simulink model "case8"  (R2024b)
settings: Solver=FixedStepAuto  StartTime=0  StopTime=1  FixedStep=1e-7  RelTol=1e-3
values from neighbouring files (symbols this model uses):
  SG_D_1_D = 0.01056    [IEEE9_case_parameters.m]    (also in case1_parameters.m; case2_parameters.m; case3_parameters.m; case4_parameters.m)
  SG_D_1_EnableSaturation = 0    [IEEE9_case_parameters.m]    (also in case1_parameters.m; case2_parameters.m; case3_parameters.m; case4_parameters.m)
  SG_D_1_f0 = 60    [IEEE9_case_parameters.m]    (also in case1_parameters.m; case2_parameters.m; case3_parameters.m; case4_parameters.m)
  SG_D_1_H = 7.5    [IEEE9_case_parameters.m]    (also in case1_parameters.m; case2_parameters.m; case3_parameters.m; case4_parameters.m)
  SG_D_1_K_A = 20    [IEEE9_case_parameters.m]    (also in case1_parameters.m; case2_parameters.m; case3_parameters.m; case4_parameters.m)
  SG_D_1_K_E = 1.000000e+1    (= 10)    [IEEE9_case_parameters.m]    (also in case1_parameters.m; case2_parameters.m; case3_parameters.m; case4_parameters.m)
  SG_D_1_K_F = 2.363    [IEEE9_case_parameters.m]    (also in case1_parameters.m; case2_parameters.m; case3_parameters.m; case4_parameters.m)
  SG_D_1_K_s = 0.5    [IEEE9_case_parameters.m]    (also in case1_parameters.m = 5; case2_parameters.m = 5; case3_parameters.m = 5; case4_parameters.m = 5)
  SG_D_1_R_a = 0.001088    [IEEE9_case_parameters.m]    (also in case1_parameters.m; case2_parameters.m; case3_parameters.m; case4_parameters.m)
  SG_D_1_S_A = 1    [IEEE9_case_parameters.m]    (also in case1_parameters.m; case2_parameters.m; case3_parameters.m; case4_parameters.m)
  SG_D_1_S_B = 0.103    [IEEE9_case_parameters.m]    (also in case1_parameters.m; case2_parameters.m; case3_parameters.m; case4_parameters.m)
  SG_D_1_S_N = 10.659857    [IEEE9_case_parameters.m]    (also in case1_parameters.m; case2_parameters.m; case3_parameters.m; case4_parameters.m)
  SG_D_1_SpeedPara = 200    [IEEE9_case_parameters.m]    (also in case1_parameters.m; case2_parameters.m; case3_parameters.m; case4_parameters.m)
  SG_D_1_T_0 = 0.720173    [IEEE9_case_parameters.m]    (also in case1_parameters.m = 0.755522; case2_parameters.m = 0.808931; case3_parameters.m = 0.869402; case4_parameters.m = 0.729316)
  SG_D_1_T_1 = 0.3    [IEEE9_case_parameters.m]    (also in case1_parameters.m; case2_parameters.m; case3_parameters.m; case4_parameters.m)
  SG_D_1_T_2 = 0.05    [IEEE9_case_parameters.m]    (also in case1_parameters.m; case2_parameters.m; case3_parameters.m; case4_parameters.m)
  SG_D_1_T_3 = 0.02    [IEEE9_case_parameters.m]    (also in case1_parameters.m; case2_parameters.m; case3_parameters.m; case4_parameters.m)
  SG_D_1_T_4 = 0.005    [IEEE9_case_parameters.m]    (also in case1_parameters.m; case2_parameters.m; case3_parameters.m; case4_parameters.m)
  SG_D_1_T_A = 0.02    [IEEE9_case_parameters.m]    (also in case1_parameters.m; case2_parameters.m; case3_parameters.m; case4_parameters.m)
  SG_D_1_T_dd = 8.000000e+0    (= 8)    [IEEE9_case_parameters.m]    (also in case1_parameters.m; case2_parameters.m; case3_parameters.m; case4_parameters.m)
  SG_D_1_T_ddd = 0.04    [IEEE9_case_parameters.m]    (also in case1_parameters.m; case2_parameters.m; case3_parameters.m; case4_parameters.m)
  SG_D_1_T_E = 0.314    [IEEE9_case_parameters.m]    (also in case1_parameters.m; case2_parameters.m; case3_parameters.m; case4_parameters.m)
  SG_D_1_T_F = 0.35    [IEEE9_case_parameters.m]    (also in case1_parameters.m; case2_parameters.m; case3_parameters.m; case4_parameters.m)
  SG_D_1_T_qd = 0.8    [IEEE9_case_parameters.m]    (also in case1_parameters.m; case2_parameters.m; case3_parameters.m; case4_parameters.m)
  SG_D_1_T_qdd = 0.02    [IEEE9_case_parameters.m]    (also in case1_parameters.m; case2_parameters.m; case3_parameters.m; case4_parameters.m)
  SG_D_1_T_speed = 0.1    [IEEE9_case_parameters.m]    (also in case1_parameters.m = 200; case2_parameters.m = 200; case3_parameters.m = 200; case4_parameters.m = 200)
  SG_D_1_T_w = 0.5    [IEEE9_case_parameters.m]    (also in case1_parameters.m; case2_parameters.m; case3_parameters.m; case4_parameters.m)
  SG_D_1_V_ref = 1.990276    [IEEE9_case_parameters.m]    (also in case1_parameters.m = 2.042296; case2_parameters.m = 2.051388; case3_parameters.m = 2.089584; case4_parameters.m = 2.01845)
  SG_D_1_w_ref = 376.991118    [IEEE9_case_parameters.m]    (also in case1_parameters.m; case2_parameters.m; case3_parameters.m; case4_parameters.m)
  SG_D_1_wb = 6.000000e+1    (= 60)    [IEEE9_case_parameters.m]    (also in case1_parameters.m; case2_parameters.m; case3_parameters.m; case4_parameters.m)
  SG_D_1_x_d = 1.9    [IEEE9_case_parameters.m]    (also in case1_parameters.m; case2_parameters.m; case3_parameters.m; case4_parameters.m)
  SG_D_1_x_dd = 0.302    [IEEE9_case_parameters.m]    (also in case1_parameters.m; case2_parameters.m; case3_parameters.m; case4_parameters.m)
  SG_D_1_x_ddd = 0.204    [IEEE9_case_parameters.m]    (also in case1_parameters.m; case2_parameters.m; case3_parameters.m; case4_parameters.m)
  SG_D_1_x_l = 0.05    [IEEE9_case_parameters.m]    (also in case1_parameters.m; case2_parameters.m; case3_parameters.m; case4_parameters.m)
  SG_D_1_x_q = 1.3    [IEEE9_case_parameters.m]    (also in case1_parameters.m; case2_parameters.m; case3_parameters.m; case4_parameters.m)
  SG_D_1_x_qd = 0.5    [IEEE9_case_parameters.m]    (also in case1_parameters.m; case2_parameters.m; case3_parameters.m; case4_parameters.m)
  SG_D_1_x_qdd = 0.3    [IEEE9_case_parameters.m]    (also in case1_parameters.m; case2_parameters.m; case3_parameters.m; case4_parameters.m)
  SG_D_2_D = 0.02    [IEEE9_case_parameters.m]    (also in case1_parameters.m; case2_parameters.m; case3_parameters.m; case4_parameters.m)
  SG_D_2_EnableSaturation = 0    [IEEE9_case_parameters.m]    (also in case1_parameters.m; case2_parameters.m; case3_parameters.m; case4_parameters.m)
  SG_D_2_f0 = 60    [IEEE9_case_parameters.m]    (also in case1_parameters.m; case2_parameters.m; case3_parameters.m; case4_parameters.m)
  SG_D_2_H = 8.000000e+0    (= 8)    [IEEE9_case_parameters.m]    (also in case1_parameters.m; case2_parameters.m; case3_parameters.m; case4_parameters.m)
  SG_D_2_K_A = 20    [IEEE9_case_parameters.m]    (also in case1_parameters.m; case2_parameters.m; case3_parameters.m; case4_parameters.m)
  SG_D_2_K_E = 1.000000e+1    (= 10)    [IEEE9_case_parameters.m]    (also in case1_parameters.m; case2_parameters.m; case3_parameters.m; case4_parameters.m)
  SG_D_2_K_F = 2.363    [IEEE9_case_parameters.m]    (also in case1_parameters.m; case2_parameters.m; case3_parameters.m; case4_parameters.m)
  SG_D_2_K_s = 0.5    [IEEE9_case_parameters.m]    (also in case1_parameters.m = 4; case2_parameters.m = 4; case3_parameters.m = 4; case4_parameters.m = 4)
  SG_D_2_R_a = 0.001088    [IEEE9_case_parameters.m]    (also in case1_parameters.m; case2_parameters.m; case3_parameters.m; case4_parameters.m)
  SG_D_2_S_A = 1    [IEEE9_case_parameters.m]    (also in case1_parameters.m; case2_parameters.m; case3_parameters.m; case4_parameters.m)
  SG_D_2_S_B = 0.103    [IEEE9_case_parameters.m]    (also in case1_parameters.m; case2_parameters.m; case3_parameters.m; case4_parameters.m)
  SG_D_2_S_N = 10.659857    [IEEE9_case_parameters.m]    (also in case1_parameters.m; case2_parameters.m; case3_parameters.m; case4_parameters.m)
  SG_D_2_SpeedPara = 200    [IEEE9_case_parameters.m]    (also in case1_parameters.m; case2_parameters.m; case3_parameters.m; case4_parameters.m)
  SG_D_2_T_0 = 1.632913    [IEEE9_case_parameters.m]    (also in case1_parameters.m = 1.632925; case2_parameters.m = 1.632915; case3_parameters.m = 1.632914; case4_parameters.m = 1.632927)
  SG_D_2_T_1 = 0.2    [IEEE9_case_parameters.m]    (also in case1_parameters.m; case2_parameters.m; case3_parameters.m; case4_parameters.m)
  SG_D_2_T_2 = 0.05    [IEEE9_case_parameters.m]    (also in case1_parameters.m; case2_parameters.m; case3_parameters.m; case4_parameters.m)
  SG_D_2_T_3 = 0.02    [IEEE9_case_parameters.m]    (also in case1_parameters.m; case2_parameters.m; case3_parameters.m; case4_parameters.m)
  SG_D_2_T_4 = 0.005    [IEEE9_case_parameters.m]    (also in case1_parameters.m; case2_parameters.m; case3_parameters.m; case4_parameters.m)
  SG_D_2_T_A = 0.02    [IEEE9_case_parameters.m]    (also in case1_parameters.m; case2_parameters.m; case3_parameters.m; case4_parameters.m)
  SG_D_2_T_dd = 7.9    [IEEE9_case_parameters.m]    (also in case1_parameters.m; case2_parameters.m; case3_parameters.m; case4_parameters.m)
  SG_D_2_T_ddd = 0.04    [IEEE9_case_parameters.m]    (also in case1_parameters.m; case2_parameters.m; case3_parameters.m; case4_parameters.m)
  SG_D_2_T_E = 0.314    [IEEE9_case_parameters.m]    (also in case1_parameters.m; case2_parameters.m; case3_parameters.m; case4_parameters.m)
  SG_D_2_T_F = 0.35    [IEEE9_case_parameters.m]    (also in case1_parameters.m; case2_parameters.m; case3_parameters.m; case4_parameters.m)
  SG_D_2_T_qd = 0.8    [IEEE9_case_parameters.m]    (also in case1_parameters.m; case2_parameters.m; case3_parameters.m; case4_parameters.m)
  SG_D_2_T_qdd = 0.015    [IEEE9_case_parameters.m]    (also in case1_parameters.m; case2_parameters.m; case3_parameters.m; case4_parameters.m)
  SG_D_2_T_speed = 0.1    [IEEE9_case_parameters.m]    (also in case1_parameters.m = 150; case2_parameters.m = 150; case3_parameters.m = 150; case4_parameters.m = 150)
  SG_D_2_T_w = 0.35    [IEEE9_case_parameters.m]    (also in case1_parameters.m; case2_parameters.m; case3_parameters.m; case4_parameters.m)
  SG_D_2_V_ref = 2.58547    [IEEE9_case_parameters.m]    (also in case1_parameters.m = 2.597896; case2_parameters.m = 2.587136; case3_parameters.m = 2.586042; case4_parameters.m = 2.599679)
  SG_D_2_w_ref = 376.991118    [IEEE9_case_parameters.m]    (also in case1_parameters.m; case2_parameters.m; case3_parameters.m; case4_parameters.m)
  SG_D_2_wb = 6.000000e+1    (= 60)    [IEEE9_case_parameters.m]    (also in case1_parameters.m; case2_parameters.m; case3_parameters.m; case4_parameters.m)
  SG_D_2_x_d = 1.8    [IEEE9_case_parameters.m]    (also in case1_parameters.m; case2_parameters.m; case3_parameters.m; case4_parameters.m)
  SG_D_2_x_dd = 0.302    [IEEE9_case_parameters.m]    (also in case1_parameters.m; case2_parameters.m; case3_parameters.m; case4_parameters.m)
  SG_D_2_x_ddd = 0.204    [IEEE9_case_parameters.m]    (also in case1_parameters.m; case2_parameters.m; case3_parameters.m; case4_parameters.m)
  SG_D_2_x_l = 0.05    [IEEE9_case_parameters.m]    (also in case1_parameters.m; case2_parameters.m; case3_parameters.m; case4_parameters.m)
  SG_D_2_x_q = 1.25    [IEEE9_case_parameters.m]    (also in case1_parameters.m; case2_parameters.m; case3_parameters.m; case4_parameters.m)
  SG_D_2_x_qd = 0.5    [IEEE9_case_parameters.m]    (also in case1_parameters.m; case2_parameters.m; case3_parameters.m; case4_parameters.m)
  SG_D_2_x_qdd = 0.3    [IEEE9_case_parameters.m]    (also in case1_parameters.m; case2_parameters.m; case3_parameters.m; case4_parameters.m)
  SG_D_3_D = 0.02    [IEEE9_case_parameters.m]    (also in case1_parameters.m; case2_parameters.m; case3_parameters.m; case4_parameters.m)
  SG_D_3_EnableSaturation = 0    [IEEE9_case_parameters.m]    (also in case1_parameters.m; case2_parameters.m; case3_parameters.m; case4_parameters.m)
  SG_D_3_f0 = 60    [IEEE9_case_parameters.m]    (also in case1_parameters.m; case2_parameters.m; case3_parameters.m; case4_parameters.m)
  SG_D_3_H = 7.7    [IEEE9_case_parameters.m]    (also in case1_parameters.m; case2_parameters.m; case3_parameters.m; case4_parameters.m)
  SG_D_3_K_A = 20    [IEEE9_case_parameters.m]    (also in case1_parameters.m; case2_parameters.m; case3_parameters.m; case4_parameters.m)
  SG_D_3_K_E = 1.000000e+1    (= 10)    [IEEE9_case_parameters.m]    (also in case1_parameters.m; case2_parameters.m; case3_parameters.m; case4_parameters.m)
  SG_D_3_K_F = 2.363    [IEEE9_case_parameters.m]    (also in case1_parameters.m; case2_parameters.m; case3_parameters.m; case4_parameters.m)
  SG_D_3_K_s = 0.2    [IEEE9_case_parameters.m]    (also in case1_parameters.m = 2; case2_parameters.m = 2; case3_parameters.m = 2; case4_parameters.m = 2)
  SG_D_3_R_a = 0.001088    [IEEE9_case_parameters.m]    (also in case1_parameters.m; case2_parameters.m; case3_parameters.m; case4_parameters.m)
  SG_D_3_S_A = 1    [IEEE9_case_parameters.m]    (also in case1_parameters.m; case2_parameters.m; case3_parameters.m; case4_parameters.m)
  SG_D_3_S_B = 0.103    [IEEE9_case_parameters.m]    (also in case1_parameters.m; case2_parameters.m; case3_parameters.m; case4_parameters.m)
  SG_D_3_S_N = 10.659857    [IEEE9_case_parameters.m]    (also in case1_parameters.m; case2_parameters.m; case3_parameters.m; case4_parameters.m)
  SG_D_3_SpeedPara = 200    [IEEE9_case_parameters.m]    (also in case1_parameters.m; case2_parameters.m; case3_parameters.m; case4_parameters.m)
  SG_D_3_T_0 = 0.850788    [IEEE9_case_parameters.m]    (also in case1_parameters.m = 0.850786; case2_parameters.m = 0.850787; case3_parameters.m; case4_parameters.m = 0.850786)
  SG_D_3_T_1 = 0.2    [IEEE9_case_parameters.m]    (also in case1_parameters.m; case2_parameters.m; case3_parameters.m; case4_parameters.m)
  SG_D_3_T_2 = 0.05    [IEEE9_case_parameters.m]    (also in case1_parameters.m; case2_parameters.m; case3_parameters.m; case4_parameters.m)
  SG_D_3_T_3 = 0.02    [IEEE9_case_parameters.m]    (also in case1_parameters.m; case2_parameters.m; case3_parameters.m; case4_parameters.m)
  SG_D_3_T_4 = 0.005    [IEEE9_case_parameters.m]    (also in case1_parameters.m; case2_parameters.m; case3_parameters.m; case4_parameters.m)
  SG_D_3_T_A = 0.02    [IEEE9_case_parameters.m]    (also in case1_parameters.m; case2_parameters.m; case3_parameters.m; case4_parameters.m)
  SG_D_3_T_dd = 8.1    [IEEE9_case_parameters.m]    (also in case1_parameters.m; case2_parameters.m; case3_parameters.m; case4_parameters.m)
  SG_D_3_T_ddd = 0.04    [IEEE9_case_parameters.m]    (also in case1_parameters.m; case2_parameters.m; case3_parameters.m; case4_parameters.m)
  SG_D_3_T_E = 0.314    [IEEE9_case_parameters.m]    (also in case1_parameters.m; case2_parameters.m; case3_parameters.m; case4_parameters.m)
  SG_D_3_T_F = 0.35    [IEEE9_case_parameters.m]    (also in case1_parameters.m; case2_parameters.m; case3_parameters.m; case4_parameters.m)
  SG_D_3_T_qd = 0.8    [IEEE9_case_parameters.m]    (also in case1_parameters.m; case2_parameters.m; case3_parameters.m; case4_parameters.m)
  SG_D_3_T_qdd = 0.015    [IEEE9_case_parameters.m]    (also in case1_parameters.m; case2_parameters.m; case3_parameters.m; case4_parameters.m)
  SG_D_3_T_speed = 0.1    [IEEE9_case_parameters.m]    (also in case1_parameters.m = 180; case2_parameters.m = 180; case3_parameters.m = 180; case4_parameters.m = 180)
  SG_D_3_T_w = 0.4    [IEEE9_case_parameters.m]    (also in case1_parameters.m; case2_parameters.m; case3_parameters.m; case4_parameters.m)
  SG_D_3_V_ref = 1.892727    [IEEE9_case_parameters.m]    (also in case1_parameters.m = 1.906439; case2_parameters.m = 1.895535; case3_parameters.m = 1.892105; case4_parameters.m = 1.906598)
  SG_D_3_w_ref = 376.991118    [IEEE9_case_parameters.m]    (also in case1_parameters.m; case2_parameters.m; case3_parameters.m; case4_parameters.m)
  SG_D_3_wb = 6.000000e+1    (= 60)    [IEEE9_case_parameters.m]    (also in case1_parameters.m; case2_parameters.m; case3_parameters.m; case4_parameters.m)
  SG_D_3_x_d = 1.85    [IEEE9_case_parameters.m]    (also in case1_parameters.m; case2_parameters.m; case3_parameters.m; case4_parameters.m)
  SG_D_3_x_dd = 0.302    [IEEE9_case_parameters.m]    (also in case1_parameters.m; case2_parameters.m; case3_parameters.m; case4_parameters.m)
  SG_D_3_x_ddd = 0.204    [IEEE9_case_parameters.m]    (also in case1_parameters.m; case2_parameters.m; case3_parameters.m; case4_parameters.m)
  SG_D_3_x_l = 0.05    [IEEE9_case_parameters.m]    (also in case1_parameters.m; case2_parameters.m; case3_parameters.m; case4_parameters.m)
  SG_D_3_x_q = 1.2    [IEEE9_case_parameters.m]    (also in case1_parameters.m; case2_parameters.m; case3_parameters.m; case4_parameters.m)
  SG_D_3_x_qd = 0.5    [IEEE9_case_parameters.m]    (also in case1_parameters.m; case2_parameters.m; case3_parameters.m; case4_parameters.m)
  SG_D_3_x_qdd = 0.3    [IEEE9_case_parameters.m]    (also in case1_parameters.m; case2_parameters.m; case3_parameters.m; case4_parameters.m)
(part 6 of 12)

== system case8/SG_D_1/d_psi_kq_SG_D_1_block ==
  note: d_psi_kq_SG_D_1 in case8
      | $-\frac{\psi _{\mathrm{gq},\mathrm{SG},D,1}+\psi _{\mathrm{kq},\mathrm{SG},D,1}+\frac{\left(x_{l}-x_{\mathrm{qd}}\right)\,\left(\psi _{q,\mathrm{SG},D,1}+\frac{\psi _{\mathrm{gq},\mathrm{SG},D,1}\,\left(x_{l}-x_{\mathrm{qdd}}\right)}{x_{l}-x_{\mathrm{qd}}}+\frac{\psi _{\mathrm{kq},\mathrm{SG},D,1}\,\left(x_{\mathrm{qd}}-x_{\mathrm{qdd}}\right)}{x_{l}-x_{\mathrm{qd}}}\right)}{x_{\mathrm{qdd}}}}{T_{\mathrm{qdd}}}$
      | Automatically generated on 2025-10-31 19:29:35 .
  State_psi_gq_SG_D_1_da5e1 : Inport
  State_psi_kq_SG_D_1_411eb : Inport  Port=2
  State_psi_gq_SG_D_1_e86a4 : Inport  Port=3
  State_psi_kq_SG_D_1_1418e : Inport  Port=4
  State_psi_q_SG_D_1_82c28 : Inport  Port=5
  Add_44a13 : Sum
  Add_4c06f : Sum
  Add_520e3 : Sum
  Add_ae062 : Sum
  Add_d3269 : Sum
  Add_e20c1 : Sum
  Constant_-1_80ff6 : Constant  Value=-1
  Constant_-1_94d95 : Constant  Value=-1
  Constant_-1_9b79f : Constant  Value=-1
  Constant_-1_c1a20 : Constant  Value=-1
  Constant_-1_d85b0 : Constant  Value=-1
  Constant_T_qdd_9f64f : Constant  Value=T_qdd
  Constant_x_l_582b3 : Constant  Value=x_l
  Constant_x_l_8869d : Constant  Value=x_l
  Constant_x_l_cf13c : Constant  Value=x_l
  Constant_x_l_d8433 : Constant  Value=x_l
  Constant_x_qd_43f7a : Constant  Value=x_qd
  Constant_x_qd_a058d : Constant  Value=x_qd
  Constant_x_qd_df308 : Constant  Value=x_qd
  Constant_x_qd_e4029 : Constant  Value=x_qd
  Constant_x_qdd_14e66 : Constant  Value=x_qdd
  Constant_x_qdd_d1b96 : Constant  Value=x_qdd
  Constant_x_qdd_f1ee5 : Constant  Value=x_qdd
  Divide_0a53e : Product  Inputs=*/
  Divide_968ff : Product  Inputs=*/
  Divide_cdea9 : Product  Inputs=*/
  Divide_e4ae6 : Product  Inputs=*/
  Product_36f02 : Product
  Product_4a984 : Product
  Product_6fe3f : Product
  Product_7e6f7 : Product
  Product_834e3 : Product
  Product_86401 : Product
  Product_9f380 : Product
  Product_cd560 : Product
  Subtract_beb8c : Sum  Inputs=+-
  Subtract_ebc89 : Sum  Inputs=+-
  Subtract_fbb2e : Sum  Inputs=+-
  Blockout_d_psi_kq_SG_D_1_0e106 : Outport
  wires:
  Product_36f02/1 -> Add_e20c1/1
  Constant_-1_80ff6/1 -> Product_36f02/1
  Constant_x_l_d8433/1 -> Product_36f02/2
  Constant_x_qdd_f1ee5/1 -> Add_e20c1/2
  Constant_-1_c1a20/1 -> Product_6fe3f/1
  Constant_x_qd_df308/1 -> Subtract_fbb2e/1
  Constant_x_qd_e4029/1 -> Add_520e3/2
  Constant_-1_d85b0/1 -> Product_4a984/1
  Constant_x_l_cf13c/1 -> Product_6fe3f/2
  Constant_x_qdd_14e66/1 -> Subtract_fbb2e/2
  Constant_x_qd_43f7a/1 -> Add_ae062/2
  Constant_x_l_582b3/1 -> Product_4a984/2
  Subtract_beb8c/1 -> Add_d3269/1
  Product_7e6f7/1 -> Subtract_beb8c/1
  State_psi_gq_SG_D_1_e86a4/1 -> Product_86401/1
  Add_e20c1/1 -> Product_86401/2
  Product_4a984/1 -> Add_4c06f/1
  Constant_x_qd_a058d/1 -> Add_4c06f/2
  State_psi_kq_SG_D_1_1418e/1 -> Product_9f380/1
  Product_6fe3f/1 -> Add_ae062/1
  Subtract_fbb2e/1 -> Product_9f380/2
  Product_86401/1 -> Divide_968ff/1
  Add_4c06f/1 -> Divide_968ff/2
  Product_9f380/1 -> Divide_0a53e/1
  Add_ae062/1 -> Divide_0a53e/2
  Constant_-1_9b79f/1 -> Product_cd560/1
  Constant_x_l_8869d/1 -> Product_cd560/2
  Divide_968ff/1 -> Subtract_ebc89/1
  Divide_0a53e/1 -> Subtract_ebc89/2
  Product_cd560/1 -> Add_520e3/1
  Add_44a13/1 -> Product_834e3/2
  Subtract_ebc89/1 -> Add_44a13/1
  State_psi_q_SG_D_1_82c28/1 -> Add_44a13/2
  Constant_-1_94d95/1 -> Product_7e6f7/1
  State_psi_gq_SG_D_1_da5e1/1 -> Product_7e6f7/2
  Divide_e4ae6/1 -> Add_d3269/2
  Product_834e3/1 -> Divide_e4ae6/1
  Add_520e3/1 -> Product_834e3/1
  State_psi_kq_SG_D_1_411eb/1 -> Subtract_beb8c/2
  Constant_x_qdd_d1b96/1 -> Divide_e4ae6/2
  Add_d3269/1 -> Divide_cdea9/1
  Constant_T_qdd_9f64f/1 -> Divide_cdea9/2
  Divide_cdea9/1 -> Blockout_d_psi_kq_SG_D_1_0e106/1

== system case8/SG_D_1/d_psi_q_SG_D_1_block ==
  note: d_psi_q_SG_D_1 in case8
      | $2\,\pi \,f_{0}\,\left(v_{d,\mathrm{SG},D,1}\,\cos\left(\theta _{\mathrm{SG},D,1}\right)+v_{q,\mathrm{SG},D,1}\,\sin\left(\theta _{\mathrm{SG},D,1}\right)-\frac{R_{a}\,\left(\psi _{q,\mathrm{SG},D,1}+\frac{\psi _{\mathrm{gq},\mathrm{SG},D,1}\,\left(x_{l}-x_{\mathrm{qdd}}\right)}{x_{l}-x_{\mathrm{qd}}}+\frac{\psi _{\mathrm{kq},\mathrm{SG},D,1}\,\left(x_{\mathrm{qd}}-x_{\mathrm{qdd}}\right)}{x_{l}-x_{\mathrm{qd}}}\right)}{x_{\mathrm{qdd}}}-\frac{\psi _{d,\mathrm{SG},D,1}\,w_{\mathrm{SG},D,1}}{2\,f_{0}\,\pi }\right)$
      | Automatically generated on 2025-10-31 19:29:30 .
  State_psi_gq_SG_D_1_7fe2e : Inport
  State_psi_kq_SG_D_1_b8294 : Inport  Port=2
  State_psi_q_SG_D_1_982cf : Inport  Port=3
  Input_v_d_SG_D_1_59a52 : Inport  Port=4
  State_theta_SG_D_1_06da5 : Inport  Port=5
  Input_v_q_SG_D_1_df1d2 : Inport  Port=6
  State_theta_SG_D_1_a61ef : Inport  Port=7
  State_psi_d_SG_D_1_9d031 : Inport  Port=8
  State_w_SG_D_1_bb027 : Inport  Port=9
  Add_5c444 : Sum
  Add_a27cd : Sum
  Add_c86fd : Sum
  Add_d6098 : Sum
  Add_ed7bc : Sum
  Constant_-1_06fe4 : Constant  Value=-1
  Constant_-1_09968 : Constant  Value=-1
  Constant_-1_faf80 : Constant  Value=-1
  Constant_-2.0_2267e : Constant  Value=-2.0
  Constant_2.0_87b9f : Constant  Value=2.0
  Constant_R_a_73440 : Constant  Value=R_a
  Constant_f0_32b31 : Constant  Value=f0
  Constant_f0_f8d6c : Constant  Value=f0
  Constant_pi_3286e : Constant  Value=pi
  Constant_pi_4e0a1 : Constant  Value=pi
  Constant_x_l_61a17 : Constant  Value=x_l
  Constant_x_l_a1f9c : Constant  Value=x_l
  Constant_x_l_f6918 : Constant  Value=x_l
  Constant_x_qd_0a3c7 : Constant  Value=x_qd
  Constant_x_qd_a448b : Constant  Value=x_qd
  Constant_x_qd_e83f7 : Constant  Value=x_qd
  Constant_x_qdd_2b385 : Constant  Value=x_qdd
  Constant_x_qdd_98a4f : Constant  Value=x_qdd
  Constant_x_qdd_9a601 : Constant  Value=x_qdd
  Divide_20893 : Product  Inputs=*/
  Divide_2ec5d : Product  Inputs=*/
  Divide_35f3f : Product  Inputs=*/
  Divide_dcf87 : Product  Inputs=*/
  MathFunc_cos_bd0e0 : Trigonometry  Operator=cos
  MathFunc_sin_a6dc1 : Trigonometry
  Product_019c9 : Product
  Product_2a58c : Product
  Product_2ca41 : Product
  Product_347ca : Product
  Product_486e4 : Product
  Product_88d0c : Product
  Product_acb5a : Product
  Product_b748f : Product
  Product_c36d3 : Product
  Product_c7bec : Product
  Product_d2a7c : Product
  Product_dd8ad : Product
  Product_eb19a : Product
  Product_ebe4b : Product
  Subtract_0ac44 : Sum  Inputs=+-
  Subtract_1ca24 : Sum  Inputs=+-
  Subtract_30cfb : Sum  Inputs=+-
  Subtract_b4afb : Sum  Inputs=+-
  Blockout_d_psi_q_SG_D_1_a9dc6 : Outport
  wires:
  Divide_35f3f/1 -> Subtract_b4afb/1
  Product_dd8ad/1 -> Add_d6098/1
  Constant_x_l_a1f9c/1 -> Product_dd8ad/2
  Constant_-1_09968/1 -> Product_dd8ad/1
  Constant_x_qdd_9a601/1 -> Add_d6098/2
  Constant_x_l_f6918/1 -> Product_2ca41/2
  Constant_-1_faf80/1 -> Product_2ca41/1
  Constant_x_l_61a17/1 -> Product_c7bec/2
  Constant_x_qdd_98a4f/1 -> Subtract_1ca24/2
  State_psi_kq_SG_D_1_b8294/1 -> Product_486e4/1
  Constant_-1_06fe4/1 -> Product_c7bec/1
  Constant_x_qd_0a3c7/1 -> Subtract_1ca24/1
  State_psi_gq_SG_D_1_7fe2e/1 -> Product_eb19a/1
  Product_347ca/1 -> Blockout_d_psi_q_SG_D_1_a9dc6/1
  Subtract_b4afb/1 -> Add_c86fd/1
  Product_eb19a/1 -> Divide_35f3f/1
  Add_d6098/1 -> Product_eb19a/2
  Divide_dcf87/1 -> Subtract_b4afb/2
  Product_2ca41/1 -> Add_ed7bc/1
  Constant_x_qd_a448b/1 -> Add_ed7bc/2
  Constant_-2.0_2267e/1 -> Product_2a58c/1
  Product_486e4/1 -> Divide_dcf87/1
  Product_c7bec/1 -> Add_a27cd/1
  Subtract_1ca24/1 -> Product_486e4/2
  Constant_x_qd_e83f7/1 -> Add_a27cd/2
  Add_ed7bc/1 -> Divide_35f3f/2
  Add_a27cd/1 -> Divide_dcf87/2
  Constant_f0_f8d6c/1 -> Product_ebe4b/2
  State_psi_q_SG_D_1_982cf/1 -> Add_c86fd/2
  Product_d2a7c/1 -> Product_c36d3/1
  Constant_R_a_73440/1 -> Product_b748f/1
  Product_c36d3/1 -> Divide_20893/2
  Product_b748f/1 -> Divide_2ec5d/1
  Add_c86fd/1 -> Product_b748f/2
  State_theta_SG_D_1_06da5/1 -> MathFunc_cos_bd0e0/1
  Input_v_d_SG_D_1_59a52/1 -> Product_019c9/1
  Constant_x_qdd_2b385/1 -> Divide_2ec5d/2
  MathFunc_cos_bd0e0/1 -> Product_019c9/2
  State_theta_SG_D_1_a61ef/1 -> MathFunc_sin_a6dc1/1
  Divide_2ec5d/1 -> Subtract_0ac44/1
  Constant_2.0_87b9f/1 -> Product_d2a7c/1
  State_w_SG_D_1_bb027/1 -> Product_acb5a/2
  Constant_pi_4e0a1/1 -> Product_d2a7c/2
  Subtract_30cfb/1 -> Add_5c444/1
  Product_019c9/1 -> Subtract_0ac44/2
  Divide_20893/1 -> Add_5c444/2
  Input_v_q_SG_D_1_df1d2/1 -> Product_88d0c/1
  MathFunc_sin_a6dc1/1 -> Product_88d0c/2
  Product_88d0c/1 -> Subtract_30cfb/2
  State_psi_d_SG_D_1_9d031/1 -> Product_acb5a/1
  Constant_f0_32b31/1 -> Product_c36d3/2
  Constant_pi_3286e/1 -> Product_2a58c/2
  Subtract_0ac44/1 -> Subtract_30cfb/1
  Product_acb5a/1 -> Divide_20893/1
  Product_2a58c/1 -> Product_ebe4b/1
  Product_ebe4b/1 -> Product_347ca/1
  Add_5c444/1 -> Product_347ca/2

== system case8/SG_D_1/d_theta_SG_D_1_block ==
  note: d_theta_SG_D_1 in case8
      | $w_{\mathrm{SG},D,1}-2\,\pi \,f_{0}$
      | Automatically generated on 2025-10-31 19:29:36 .
  State_w_SG_D_1_1d023 : Inport
  Add_d6c34 : Sum
  Constant_-2.0_1c6c2 : Constant  Value=-2.0
  Constant_f0_3bb0f : Constant  Value=f0
  Constant_pi_2d319 : Constant  Value=pi
  Product_4123a : Product
  Product_fbd34 : Product
  Blockout_d_theta_SG_D_1_4230e : Outport
  wires:
  State_w_SG_D_1_1d023/1 -> Add_d6c34/2
  Constant_-2.0_1c6c2/1 -> Product_4123a/1
  Constant_f0_3bb0f/1 -> Product_fbd34/2
  Constant_pi_2d319/1 -> Product_4123a/2
  Product_fbd34/1 -> Add_d6c34/1
  Product_4123a/1 -> Product_fbd34/1
  Add_d6c34/1 -> Blockout_d_theta_SG_D_1_4230e/1

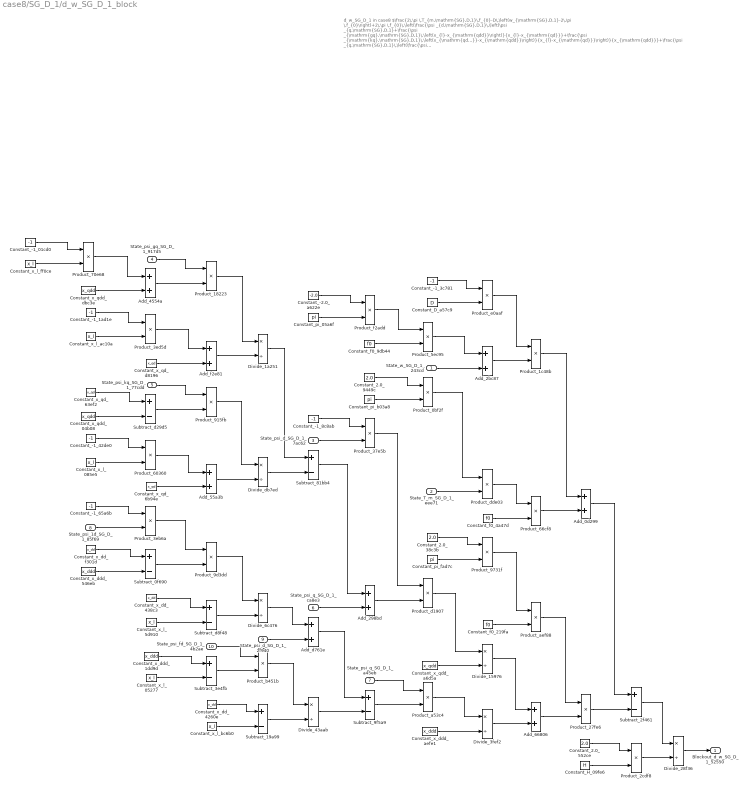
== system case8/SG_D_1/d_w_SG_D_1_block ==
  note: d_w_SG_D_1 in case8
      | $\frac{2\,\pi \,T_{m,\mathrm{SG},D,1}\,f_{0}-D\,\left(w_{\mathrm{SG},D,1}-2\,\pi \,f_{0}\right)+2\,\pi \,f_{0}\,\left(\frac{\psi _{d,\mathrm{SG},D,1}\,\left(\psi _{q,\mathrm{SG},D,1}+\frac{\psi _{\mathrm{gq},\mathrm{SG},D,1}\,\left(x_{l}-x_{\mathrm{qdd}}\right)}{x_{l}-x_{\mathrm{qd}}}+\frac{\psi _{\mathrm{kq},\mathrm{SG},D,1}\,\left(x_{\mathrm{qd}}-x_{\mathrm{qdd}}\right)}{x_{l}-x_{\mathrm{qd}}}\right)}{x_{\mathrm{qdd}}}+\frac{\psi _{q,\mathrm{SG},D,1}\,\left(\frac{\psi _{\mathrm{1d},\mathrm{SG},D,1}\,\left(x_{\mathrm{dd}}-x_{\mathrm{ddd}}\right)}{x_{\mathrm{dd}}-x_{l}}-\psi _{d,\mathrm{SG},D,1}+\frac{\psi _{\mathrm{fd},\mathrm{SG},D,1}\,\left(x_{\mathrm{ddd}}-x_{l}\right)}{x_{\mathrm{dd}}-x_{l}}\right)}{x_{\mathrm{ddd}}}\right)}{2\,H}$
      | Automatically generated on 2025-10-31 19:29:36 .
  State_w_SG_D_1_243cd : Inport
  State_T_m_SG_D_1_eee71 : Inport  Port=2
  State_psi_d_SG_D_1_7ac62 : Inport  Port=3
  State_psi_gq_SG_D_1_917d5 : Inport  Port=4
  State_psi_kq_SG_D_1_77cdd : Inport  Port=5
  State_psi_q_SG_D_1_ca8e3 : Inport  Port=6
  State_psi_q_SG_D_1_a45eb : Inport  Port=7
  State_psi_1d_SG_D_1_85f69 : Inport  Port=8
  State_psi_d_SG_D_1_2f940 : Inport  Port=9
  State_psi_fd_SG_D_1_4b2ae : Inport  Port=10
  Add_0d299 : Sum
  Add_298bd : Sum
  Add_2bc87 : Sum
  Add_4554a : Sum
  Add_55a3b : Sum
  Add_66806 : Sum
  Add_d761e : Sum
  Add_f2e81 : Sum
  Constant_-1_01cd0 : Constant  Value=-1
  Constant_-1_1ad1e : Constant  Value=-1
  Constant_-1_3c781 : Constant  Value=-1
  Constant_-1_42de0 : Constant  Value=-1
  Constant_-1_65a6b : Constant  Value=-1
  Constant_-1_8c8ab : Constant  Value=-1
  Constant_-2.0_a622e : Constant  Value=-2.0
  Constant_2.0_38c3b : Constant  Value=2.0
  Constant_2.0_552ce : Constant  Value=2.0
  Constant_2.0_9449c : Constant  Value=2.0
  Constant_D_a57c9 : Constant  Value=D
  Constant_H_09fe6 : Constant  Value=H
  Constant_f0_219fa : Constant  Value=f0
  Constant_f0_4a47d : Constant  Value=f0
  Constant_f0_9db44 : Constant  Value=f0
  Constant_pi_05a6f : Constant  Value=pi
  Constant_pi_b03a8 : Constant  Value=pi
  Constant_pi_fad7c : Constant  Value=pi
  Constant_x_dd_4260e : Constant  Value=x_dd
  Constant_x_dd_438c3 : Constant  Value=x_dd
  Constant_x_dd_f301d : Constant  Value=x_dd
  Constant_x_ddd_1dd9d : Constant  Value=x_ddd
  Constant_x_ddd_546eb : Constant  Value=x_ddd
  Constant_x_ddd_aefe1 : Constant  Value=x_ddd
  Constant_x_l_05277 : Constant  Value=x_l
  Constant_x_l_085e5 : Constant  Value=x_l
  Constant_x_l_5d910 : Constant  Value=x_l
  Constant_x_l_ac10a : Constant  Value=x_l
  Constant_x_l_bc6b0 : Constant  Value=x_l
  Constant_x_l_ff0ce : Constant  Value=x_l
  Constant_x_qd_63ef2 : Constant  Value=x_qd
  Constant_x_qd_6b94e : Constant  Value=x_qd
  Constant_x_qd_d8196 : Constant  Value=x_qd
  Constant_x_qdd_04b08 : Constant  Value=x_qdd
  Constant_x_qdd_a6d5a : Constant  Value=x_qdd
  Constant_x_qdd_dbc3e : Constant  Value=x_qdd
  Divide_15976 : Product  Inputs=*/
  Divide_1a251 : Product  Inputs=*/
  Divide_28f36 : Product  Inputs=*/
  Divide_3fef2 : Product  Inputs=*/
  Divide_43aab : Product  Inputs=*/
  Divide_6c476 : Product  Inputs=*/
  Divide_db7ed : Product  Inputs=*/
  Product_0bf2f : Product
  Product_18223 : Product
  Product_1c48b : Product
  Product_27fe6 : Product
  Product_2cdf8 : Product
  Product_37e5b : Product
  Product_3eb6a : Product
  Product_3ed5d : Product
  Product_5ec95 : Product
  Product_60360 : Product
  Product_66cf8 : Product
  Product_70e68 : Product
  Product_915fb : Product
  Product_9731f : Product
  Product_9d3dd : Product
  Product_a53c4 : Product
  Product_aef88 : Product
  Product_b451b : Product
  Product_d1907 : Product
  Product_dde03 : Product
  Product_e0aaf : Product
  Product_f2add : Product
  Subtract_0f690 : Sum  Inputs=+-
  Subtract_19a99 : Sum  Inputs=+-
  Subtract_2f461 : Sum  Inputs=+-
  Subtract_3e4fb : Sum  Inputs=+-
  Subtract_81bb4 : Sum  Inputs=+-
  Subtract_9f5a9 : Sum  Inputs=+-
  Subtract_d29d5 : Sum  Inputs=+-
  Subtract_d8f48 : Sum  Inputs=+-
  Blockout_d_w_SG_D_1_52550 : Outport
  wires:
  Product_5ec95/1 -> Add_2bc87/1
  Constant_-1_01cd0/1 -> Product_70e68/1
  Constant_pi_b03a8/1 -> Product_0bf2f/2
  Constant_x_qdd_dbc3e/1 -> Add_4554a/2
  Constant_x_l_ff0ce/1 -> Product_70e68/2
  Product_70e68/1 -> Add_4554a/1
  Constant_x_qd_63ef2/1 -> Subtract_d29d5/1
  Constant_-1_1ad1e/1 -> Product_3ed5d/1
  Product_f2add/1 -> Product_5ec95/1
  Constant_x_qdd_04b08/1 -> Subtract_d29d5/2
  State_psi_q_SG_D_1_a45eb/1 -> Product_a53c4/1
  Constant_x_l_ac10a/1 -> Product_3ed5d/2
  Constant_-1_42de0/1 -> Product_60360/1
  Constant_x_l_085e5/1 -> Product_60360/2
  Constant_-1_65a6b/1 -> Product_3eb6a/1
  Product_3ed5d/1 -> Add_f2e81/1
  State_psi_1d_SG_D_1_85f69/1 -> Product_3eb6a/2
  Constant_x_dd_f301d/1 -> Subtract_0f690/1
  Subtract_d29d5/1 -> Product_915fb/2
  Constant_x_ddd_546eb/1 -> Subtract_0f690/2
  State_psi_gq_SG_D_1_917d5/1 -> Product_18223/1
  Product_37e5b/1 -> Product_d1907/1
  Add_4554a/1 -> Product_18223/2
  Constant_x_qd_d8196/1 -> Add_f2e81/2
  State_psi_kq_SG_D_1_77cdd/1 -> Product_915fb/1
  Constant_f0_9db44/1 -> Product_5ec95/2
  Product_60360/1 -> Add_55a3b/1
  Constant_x_dd_438c3/1 -> Subtract_d8f48/1
  Constant_x_qd_6b94e/1 -> Add_55a3b/2
  Product_3eb6a/1 -> Product_9d3dd/1
  Subtract_0f690/1 -> Product_9d3dd/2
  Constant_x_l_5d910/1 -> Subtract_d8f48/2
  Constant_x_ddd_1dd9d/1 -> Subtract_3e4fb/1
  Constant_x_l_05277/1 -> Subtract_3e4fb/2
  State_w_SG_D_1_243cd/1 -> Add_2bc87/2
  Divide_15976/1 -> Add_66806/1
  Constant_-1_3c781/1 -> Product_e0aaf/1
  Product_18223/1 -> Divide_1a251/1
  Add_2bc87/1 -> Product_1c48b/2
  Divide_1a251/1 -> Subtract_81bb4/1
  Add_f2e81/1 -> Divide_1a251/2
  Constant_pi_05a6f/1 -> Product_f2add/2
  Product_915fb/1 -> Divide_db7ed/1
  Add_55a3b/1 -> Divide_db7ed/2
  Product_9d3dd/1 -> Divide_6c476/1
  Divide_6c476/1 -> Add_d761e/1
  Subtract_d8f48/1 -> Divide_6c476/2
  State_psi_fd_SG_D_1_4b2ae/1 -> Product_b451b/1
  Subtract_3e4fb/1 -> Product_b451b/2
  Constant_x_dd_4260e/1 -> Subtract_19a99/1
  Constant_x_l_bc6b0/1 -> Subtract_19a99/2
  Divide_db7ed/1 -> Subtract_81bb4/2
  Constant_2.0_9449c/1 -> Product_0bf2f/1
  State_psi_d_SG_D_1_2f940/1 -> Add_d761e/2
  Product_b451b/1 -> Divide_43aab/1
  Subtract_19a99/1 -> Divide_43aab/2
  Constant_-2.0_a622e/1 -> Product_f2add/1
  Constant_-1_8c8ab/1 -> Product_37e5b/1
  State_psi_d_SG_D_1_7ac62/1 -> Product_37e5b/2
  Subtract_81bb4/1 -> Add_298bd/1
  Subtract_9f5a9/1 -> Product_a53c4/2
  State_psi_q_SG_D_1_ca8e3/1 -> Add_298bd/2
  Add_d761e/1 -> Subtract_9f5a9/1
  Divide_43aab/1 -> Subtract_9f5a9/2
  Add_298bd/1 -> Product_d1907/2
  Constant_D_a57c9/1 -> Product_e0aaf/2
  Product_0bf2f/1 -> Product_dde03/1
  State_T_m_SG_D_1_eee71/1 -> Product_dde03/2
  Constant_2.0_38c3b/1 -> Product_9731f/1
  Constant_pi_fad7c/1 -> Product_9731f/2
  Product_d1907/1 -> Divide_15976/1
  Constant_x_qdd_a6d5a/1 -> Divide_15976/2
  Product_a53c4/1 -> Divide_3fef2/1
  Constant_x_ddd_aefe1/1 -> Divide_3fef2/2
  Product_e0aaf/1 -> Product_1c48b/1
  Product_dde03/1 -> Product_66cf8/1
  Constant_f0_4a47d/1 -> Product_66cf8/2
  Product_9731f/1 -> Product_aef88/1
  Constant_f0_219fa/1 -> Product_aef88/2
  Divide_3fef2/1 -> Add_66806/2
  Product_1c48b/1 -> Add_0d299/1
  Product_66cf8/1 -> Add_0d299/2
  Product_aef88/1 -> Product_27fe6/1
  Add_66806/1 -> Product_27fe6/2
  Add_0d299/1 -> Subtract_2f461/1
  Product_27fe6/1 -> Subtract_2f461/2
  Constant_2.0_552ce/1 -> Product_2cdf8/1
  Constant_H_09fe6/1 -> Product_2cdf8/2
  Subtract_2f461/1 -> Divide_28f36/1
  Product_2cdf8/1 -> Divide_28f36/2
  Divide_28f36/1 -> Blockout_d_w_SG_D_1_52550/1

== system case8/SG_D_1/i_d_SG_D_1_block ==
  note: i_d_SG_D_1 in case8
      | $\frac{\sin\left(\theta _{\mathrm{SG},D,1}\right)\,\left(\frac{\psi _{\mathrm{1d},\mathrm{SG},D,1}\,\left(x_{\mathrm{dd}}-x_{\mathrm{ddd}}\right)}{x_{\mathrm{dd}}-x_{l}}-\psi _{d,\mathrm{SG},D,1}+\frac{\psi _{\mathrm{fd},\mathrm{SG},D,1}\,\left(x_{\mathrm{ddd}}-x_{l}\right)}{x_{\mathrm{dd}}-x_{l}}\right)}{x_{\mathrm{ddd}}}-\frac{\cos\left(\theta _{\mathrm{SG},D,1}\right)\,\left(\psi _{q,\mathrm{SG},D,1}+\frac{\psi _{\mathrm{gq},\mathrm{SG},D,1}\,\left(x_{l}-x_{\mathrm{qdd}}\right)}{x_{l}-x_{\mathrm{qd}}}+\frac{\psi _{\mathrm{kq},\mathrm{SG},D,1}\,\left(x_{\mathrm{qd}}-x_{\mathrm{qdd}}\right)}{x_{l}-x_{\mathrm{qd}}}\right)}{x_{\mathrm{qdd}}}$
      | Automatically generated on 2025-10-31 19:29:41 .
  State_psi_gq_SG_D_1_b21d8 : Inport
  State_psi_kq_SG_D_1_f4c63 : Inport  Port=2
  State_psi_q_SG_D_1_4cfdc : Inport  Port=3
  State_theta_SG_D_1_5398a : Inport  Port=4
  State_psi_1d_SG_D_1_b5c8c : Inport  Port=5
  State_psi_d_SG_D_1_e1c0f : Inport  Port=6
  State_psi_fd_SG_D_1_12327 : Inport  Port=7
  State_theta_SG_D_1_01785 : Inport  Port=8
  Add_09c57 : Sum
  Add_25983 : Sum
  Add_8205d : Sum
  Add_abafd : Sum
  Add_be2c2 : Sum
  Constant_-1_1707f : Constant  Value=-1
  Constant_-1_1a3c8 : Constant  Value=-1
  Constant_-1_3341b : Constant  Value=-1
  Constant_-1_8c8cd : Constant  Value=-1
  Constant_-1_e4d56 : Constant  Value=-1
  Constant_x_dd_138ae : Constant  Value=x_dd
  Constant_x_dd_33679 : Constant  Value=x_dd
  Constant_x_dd_dae60 : Constant  Value=x_dd
  Constant_x_ddd_13a77 : Constant  Value=x_ddd
  Constant_x_ddd_99981 : Constant  Value=x_ddd
  Constant_x_ddd_f56ae : Constant  Value=x_ddd
  Constant_x_l_06963 : Constant  Value=x_l
  Constant_x_l_60759 : Constant  Value=x_l
  Constant_x_l_75983 : Constant  Value=x_l
  Constant_x_l_84dec : Constant  Value=x_l
  Constant_x_l_87258 : Constant  Value=x_l
  Constant_x_l_b2b7b : Constant  Value=x_l
  Constant_x_qd_42108 : Constant  Value=x_qd
  Constant_x_qd_85a60 : Constant  Value=x_qd
  Constant_x_qd_fb30a : Constant  Value=x_qd
  Constant_x_qdd_06c33 : Constant  Value=x_qdd
  Constant_x_qdd_543a1 : Constant  Value=x_qdd
  Constant_x_qdd_cf3b3 : Constant  Value=x_qdd
  Divide_72a62 : Product  Inputs=*/
  Divide_820be : Product  Inputs=*/
  Divide_91525 : Product  Inputs=*/
  Divide_ab51a : Product  Inputs=*/
  Divide_eb233 : Product  Inputs=*/
  Divide_ff27e : Product  Inputs=*/
  MathFunc_cos_ae8be : Trigonometry  Operator=cos
  MathFunc_sin_1a7aa : Trigonometry
  Product_25f2c : Product
  Product_38d5c : Product
  Product_3cdba : Product
  Product_4fc31 : Product
  Product_5b3c2 : Product
  Product_bf093 : Product
  Product_cba09 : Product
  Product_cda70 : Product
  Product_d7085 : Product
  Product_e9607 : Product
  Product_fc543 : Product
  Subtract_00c70 : Sum  Inputs=+-
  Subtract_1c49f : Sum  Inputs=+-
  Subtract_1ecc0 : Sum  Inputs=+-
  Subtract_4499d : Sum  Inputs=+-
  Subtract_89811 : Sum  Inputs=+-
  Subtract_91f5e : Sum  Inputs=+-
  Subtract_b6760 : Sum  Inputs=+-
  Subtract_fd651 : Sum  Inputs=+-
  Blockout_i_d_SG_D_1_dfa0a : Outport
  wires:
  Constant_-1_e4d56/1 -> Product_fc543/1
  Constant_x_l_87258/1 -> Product_fc543/2
  Constant_x_ddd_13a77/1 -> Subtract_89811/2
  Product_fc543/1 -> Add_8205d/1
  Constant_x_qdd_543a1/1 -> Subtract_4499d/2
  Constant_x_l_60759/1 -> Product_e9607/2
  Constant_x_qd_fb30a/1 -> Add_09c57/2
  Constant_x_qdd_cf3b3/1 -> Add_8205d/2
  Constant_x_qd_85a60/1 -> Subtract_4499d/1
  MathFunc_cos_ae8be/1 -> Product_cba09/2
  Constant_-1_3341b/1 -> Product_e9607/1
  Constant_-1_8c8cd/1 -> Product_25f2c/1
  Subtract_1ecc0/1 -> Blockout_i_d_SG_D_1_dfa0a/1
  Constant_x_l_75983/1 -> Product_25f2c/2
  Divide_eb233/1 -> Subtract_00c70/1
  State_psi_gq_SG_D_1_b21d8/1 -> Product_4fc31/1
  Subtract_91f5e/1 -> Product_cda70/2
  Add_8205d/1 -> Product_4fc31/2
  Divide_820be/1 -> Add_be2c2/1
  Product_e9607/1 -> Add_25983/1
  Constant_x_qd_42108/1 -> Add_25983/2
  State_psi_kq_SG_D_1_f4c63/1 -> Product_bf093/1
  Add_be2c2/1 -> Subtract_b6760/1
  Add_25983/1 -> Divide_eb233/2
  Subtract_4499d/1 -> Product_bf093/2
  Product_25f2c/1 -> Add_09c57/1
  Constant_-1_1707f/1 -> Product_38d5c/1
  State_psi_1d_SG_D_1_b5c8c/1 -> Product_38d5c/2
  Constant_x_dd_dae60/1 -> Subtract_89811/1
  Product_4fc31/1 -> Divide_eb233/1
  Product_5b3c2/1 -> Divide_ff27e/1
  Subtract_89811/1 -> Product_d7085/2
  Product_bf093/1 -> Divide_72a62/1
  Product_38d5c/1 -> Product_d7085/1
  Add_09c57/1 -> Divide_72a62/2
  Constant_x_dd_33679/1 -> Subtract_fd651/1
  Subtract_00c70/1 -> Add_abafd/1
  Constant_x_l_84dec/1 -> Subtract_fd651/2
  Constant_x_ddd_f56ae/1 -> Subtract_91f5e/1
  Constant_x_l_b2b7b/1 -> Subtract_91f5e/2
  Divide_ff27e/1 -> Subtract_1ecc0/2
  Divide_72a62/1 -> Subtract_00c70/2
  State_theta_SG_D_1_5398a/1 -> MathFunc_cos_ae8be/1
  Product_d7085/1 -> Divide_820be/1
  Subtract_fd651/1 -> Divide_820be/2
  State_theta_SG_D_1_01785/1 -> MathFunc_sin_1a7aa/1
  State_psi_fd_SG_D_1_12327/1 -> Product_cda70/1
  Constant_x_dd_138ae/1 -> Subtract_1c49f/1
  Constant_x_l_06963/1 -> Subtract_1c49f/2
  State_psi_q_SG_D_1_4cfdc/1 -> Add_abafd/2
  State_psi_d_SG_D_1_e1c0f/1 -> Add_be2c2/2
  Constant_x_ddd_99981/1 -> Divide_ff27e/2
  MathFunc_sin_1a7aa/1 -> Product_5b3c2/2
  Product_cda70/1 -> Divide_ab51a/1
  Constant_-1_1a3c8/1 -> Product_3cdba/1
  Subtract_1c49f/1 -> Divide_ab51a/2
  Add_abafd/1 -> Product_3cdba/2
  Divide_ab51a/1 -> Subtract_b6760/2
  Product_3cdba/1 -> Product_cba09/1
  Subtract_b6760/1 -> Product_5b3c2/1
  Constant_x_qdd_06c33/1 -> Divide_91525/2
  Product_cba09/1 -> Divide_91525/1
  Divide_91525/1 -> Subtract_1ecc0/1

== system case8/SG_D_1/i_q_SG_D_1_block ==
  note: i_q_SG_D_1 in case8
      | $-\frac{\sin\left(\theta _{\mathrm{SG},D,1}\right)\,\left(\psi _{q,\mathrm{SG},D,1}+\frac{\psi _{\mathrm{gq},\mathrm{SG},D,1}\,\left(x_{l}-x_{\mathrm{qdd}}\right)}{x_{l}-x_{\mathrm{qd}}}+\frac{\psi _{\mathrm{kq},\mathrm{SG},D,1}\,\left(x_{\mathrm{qd}}-x_{\mathrm{qdd}}\right)}{x_{l}-x_{\mathrm{qd}}}\right)}{x_{\mathrm{qdd}}}-\frac{\cos\left(\theta _{\mathrm{SG},D,1}\right)\,\left(\frac{\psi _{\mathrm{1d},\mathrm{SG},D,1}\,\left(x_{\mathrm{dd}}-x_{\mathrm{ddd}}\right)}{x_{\mathrm{dd}}-x_{l}}-\psi _{d,\mathrm{SG},D,1}+\frac{\psi _{\mathrm{fd},\mathrm{SG},D,1}\,\left(x_{\mathrm{ddd}}-x_{l}\right)}{x_{\mathrm{dd}}-x_{l}}\right)}{x_{\mathrm{ddd}}}$
      | Automatically generated on 2025-10-31 19:29:42 .
  State_psi_gq_SG_D_1_7cf70 : Inport
  State_psi_kq_SG_D_1_e7e60 : Inport  Port=2
  State_psi_q_SG_D_1_51331 : Inport  Port=3
  State_theta_SG_D_1_65208 : Inport  Port=4
  State_psi_1d_SG_D_1_b3786 : Inport  Port=5
  State_psi_d_SG_D_1_80107 : Inport  Port=6
  State_psi_fd_SG_D_1_87650 : Inport  Port=7
  State_theta_SG_D_1_ba088 : Inport  Port=8
  Add_0194a : Sum
  Add_494f7 : Sum
  Add_71b67 : Sum
  Add_80ada : Sum
  Add_90f2b : Sum
  Add_a5200 : Sum
  Constant_-1_1963f : Constant  Value=-1
  Constant_-1_2de7f : Constant  Value=-1
  Constant_-1_535ce : Constant  Value=-1
  Constant_-1_c8c4a : Constant  Value=-1
  Constant_-1_ccc6a : Constant  Value=-1
  Constant_x_dd_0ae51 : Constant  Value=x_dd
  Constant_x_dd_ab82e : Constant  Value=x_dd
  Constant_x_dd_f0a6a : Constant  Value=x_dd
  Constant_x_ddd_13b30 : Constant  Value=x_ddd
  Constant_x_ddd_e29f2 : Constant  Value=x_ddd
  Constant_x_ddd_ee067 : Constant  Value=x_ddd
  Constant_x_l_45a53 : Constant  Value=x_l
  Constant_x_l_5f2ca : Constant  Value=x_l
  Constant_x_l_a4925 : Constant  Value=x_l
  Constant_x_l_c03f7 : Constant  Value=x_l
  Constant_x_l_d7c16 : Constant  Value=x_l
  Constant_x_l_ecd51 : Constant  Value=x_l
  Constant_x_qd_77415 : Constant  Value=x_qd
  Constant_x_qd_8f5cf : Constant  Value=x_qd
  Constant_x_qd_ed096 : Constant  Value=x_qd
  Constant_x_qdd_20720 : Constant  Value=x_qdd
  Constant_x_qdd_2f1d5 : Constant  Value=x_qdd
  Constant_x_qdd_c1b32 : Constant  Value=x_qdd
  Divide_11d4d : Product  Inputs=*/
  Divide_3cd76 : Product  Inputs=*/
  Divide_60a96 : Product  Inputs=*/
  Divide_98f29 : Product  Inputs=*/
  Divide_ae8cb : Product  Inputs=*/
  Divide_c51e2 : Product  Inputs=*/
  MathFunc_cos_d6572 : Trigonometry  Operator=cos
  MathFunc_sin_e99e6 : Trigonometry
  Product_144e1 : Product
  Product_21b94 : Product
  Product_25db7 : Product
  Product_44bbb : Product
  Product_63782 : Product
  Product_7a754 : Product
  Product_b7c8d : Product
  Product_c7dfd : Product
  Product_e8841 : Product
  Product_ef3a0 : Product
  Product_fbc37 : Product
  Subtract_14cf2 : Sum  Inputs=+-
  Subtract_5571b : Sum  Inputs=+-
  Subtract_5eca2 : Sum  Inputs=+-
  Subtract_84239 : Sum  Inputs=+-
  Subtract_c9030 : Sum  Inputs=+-
  Subtract_de3a2 : Sum  Inputs=+-
  Subtract_f89ab : Sum  Inputs=+-
  Blockout_i_q_SG_D_1_34308 : Outport
  wires:
  State_theta_SG_D_1_ba088/1 -> MathFunc_cos_d6572/1
  State_psi_fd_SG_D_1_87650/1 -> Product_63782/1
  Constant_-1_2de7f/1 -> Product_b7c8d/1
  Constant_x_l_5f2ca/1 -> Product_b7c8d/2
  Subtract_84239/1 -> Product_63782/2
  Constant_x_l_d7c16/1 -> Subtract_f89ab/2
  Product_b7c8d/1 -> Add_80ada/1
  Constant_x_qdd_20720/1 -> Add_80ada/2
  Constant_x_qd_8f5cf/1 -> Subtract_5eca2/1
  Constant_x_qdd_c1b32/1 -> Divide_3cd76/2
  MathFunc_sin_e99e6/1 -> Product_44bbb/2
  Constant_-1_1963f/1 -> Product_21b94/1
  Constant_x_qdd_2f1d5/1 -> Subtract_5eca2/2
  Add_90f2b/1 -> Product_e8841/2
  Product_144e1/1 -> Divide_60a96/1
  Constant_x_l_c03f7/1 -> Product_21b94/2
  Constant_-1_ccc6a/1 -> Product_c7dfd/1
  Constant_x_l_ecd51/1 -> Product_c7dfd/2
  State_psi_gq_SG_D_1_7cf70/1 -> Product_144e1/1
  Add_80ada/1 -> Product_144e1/2
  Divide_98f29/1 -> Add_0194a/1
  Product_21b94/1 -> Add_71b67/1
  Divide_3cd76/1 -> Add_494f7/1
  Constant_x_qd_ed096/1 -> Add_71b67/2
  State_psi_kq_SG_D_1_e7e60/1 -> Product_fbc37/1
  Add_0194a/1 -> Subtract_de3a2/1
  Subtract_5eca2/1 -> Product_fbc37/2
  Divide_60a96/1 -> Subtract_c9030/1
  Add_71b67/1 -> Divide_60a96/2
  Product_c7dfd/1 -> Add_a5200/1
  Constant_x_qd_77415/1 -> Add_a5200/2
  Constant_-1_535ce/1 -> Product_7a754/1
  MathFunc_cos_d6572/1 -> Product_25db7/2
  Product_63782/1 -> Divide_11d4d/1
  State_psi_1d_SG_D_1_b3786/1 -> Product_7a754/2
  Constant_x_l_45a53/1 -> Subtract_5571b/2
  Constant_x_dd_ab82e/1 -> Subtract_14cf2/1
  Divide_11d4d/1 -> Subtract_de3a2/2
  Constant_x_ddd_ee067/1 -> Subtract_14cf2/2
  Product_25db7/1 -> Divide_ae8cb/1
  Product_fbc37/1 -> Divide_c51e2/1
  Product_7a754/1 -> Product_ef3a0/1
  Add_a5200/1 -> Divide_c51e2/2
  Subtract_14cf2/1 -> Product_ef3a0/2
  State_psi_d_SG_D_1_80107/1 -> Add_0194a/2
  Constant_x_dd_f0a6a/1 -> Subtract_f89ab/1
  Constant_x_ddd_e29f2/1 -> Subtract_84239/1
  Constant_x_l_a4925/1 -> Subtract_84239/2
  Divide_ae8cb/1 -> Add_494f7/2
  Divide_c51e2/1 -> Subtract_c9030/2
  State_theta_SG_D_1_65208/1 -> MathFunc_sin_e99e6/1
  Product_ef3a0/1 -> Divide_98f29/1
  Subtract_f89ab/1 -> Divide_98f29/2
  Constant_x_dd_0ae51/1 -> Subtract_5571b/1
  Subtract_c9030/1 -> Add_90f2b/1
  State_psi_q_SG_D_1_51331/1 -> Add_90f2b/2
  Subtract_5571b/1 -> Divide_11d4d/2
  Subtract_de3a2/1 -> Product_25db7/1
  Constant_-1_c8c4a/1 -> Product_e8841/1
  Product_e8841/1 -> Product_44bbb/1
  Product_44bbb/1 -> Divide_3cd76/1
  Constant_x_ddd_13b30/1 -> Divide_ae8cb/2
  Add_494f7/1 -> Blockout_i_q_SG_D_1_34308/1

== system case8/SG_D_1/theta_SG_D_1_out_block ==
  note: theta_SG_D_1_out in case8
      | $\theta _{\mathrm{SG},D,1}$
      | Automatically generated on 2025-10-31 19:29:43 .
  State_theta_SG_D_1_6aa7c : Inport
  Blockout_theta_SG_D_1_out_3488a : Outport
  wires:
  State_theta_SG_D_1_6aa7c/1 -> Blockout_theta_SG_D_1_out_3488a/1

== system case8/SG_D_1/w_SG_D_1_out_block ==
  note: w_SG_D_1_out in case8
      | $w_{\mathrm{SG},D,1}$
      | Automatically generated on 2025-10-31 19:29:43 .
  State_w_SG_D_1_9c2ee : Inport
  Blockout_w_SG_D_1_out_685b6 : Outport
  wires:
  State_w_SG_D_1_9c2ee/1 -> Blockout_w_SG_D_1_out_685b6/1
